simulink model "Control_Block_2021"  (R2022a)
settings: Solver=FixedStepAuto  StartTime=0.0  StopTime=end_time  FixedStep=dt  RelTol=1e-3
values from neighbouring files (symbols this model uses):
  Area = pi() * r0^2    [Main_PD_Control.m]    (also in Test_code.m; main.m = 1.25663706144e-05; main2.m = 1.25663706144e-05)
  Cd = 0.42    [Main_PD_Control.m]    (also in Test_code.m; main.m = 1.05; main2.m = 1.05)
  dl = l / (N - 1)    (= 0.0102040816327)    [load_parameter.m]    (also in main.m; main2.m; testcode_2d.m = 0.0204081632653)
  dt = 0.01    [Main_PD_Control.m]    (also in Test_code.m; load_parameter.m; main.m; main2.m = 0.001)
  EA = E*A    (= 13.8544236023)    [load_parameter.m]    (also in main.m; main2.m; testcode_2d.m = 10555751.3161)
  EI = E*I    (= 1.73180295029e-05)    [load_parameter.m]    (also in main.m; main2.m; testcode_2d.m = 765.291970414)
  K_d = 10    [Main_PD_Control.m]    (also in Test_code.m = 0; main.m; main2.m)
  K_p = 100    [Main_PD_Control.m]    (also in Test_code.m; main.m = 500; main2.m)
  M = zeros(2*N,2*N)    [load_parameter.m]    (also in main.m; main2.m; testcode_2d.m)
  N = length(old_posi)/2    [BoundryJudge.m]    (also in load_parameter.m = 50; main.m = 50; main2.m = 50; testcode_2d.m = 50)
  q0 = zeros(2*N,1)    [load_parameter.m]    (also in main.m; main2.m; testcode_2d.m = q)
  rho_blood = 1025    [main.m]    (also in main2.m)
  tol = EI / l^2 * 1e-3    (= 6.92721180117e-08)    [load_parameter.m]    (also in main.m; main2.m; testcode_2d.m = 0.765291970414)
settings Model: Creator=zhong  LastModifiedBy=zhong
settings DebuggingCC: UnconnectedInputMsg=warning  UnconnectedOutputMsg=warning  UnconnectedLineMsg=warning  UnderSpecifiedDimensionMsg=error
settings RTWCC: DLArmComputeVersion=19.05

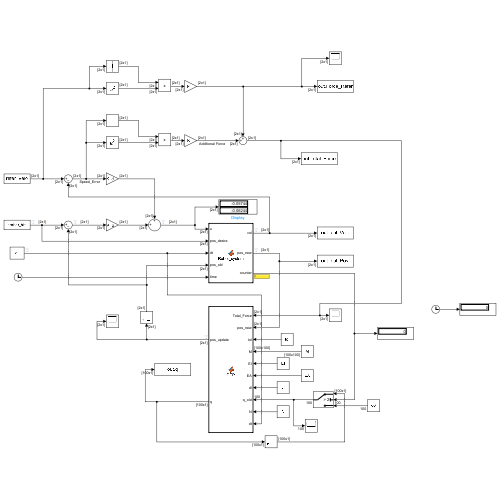
[thumbnail: Simulink's stored preview of the top-level diagram]
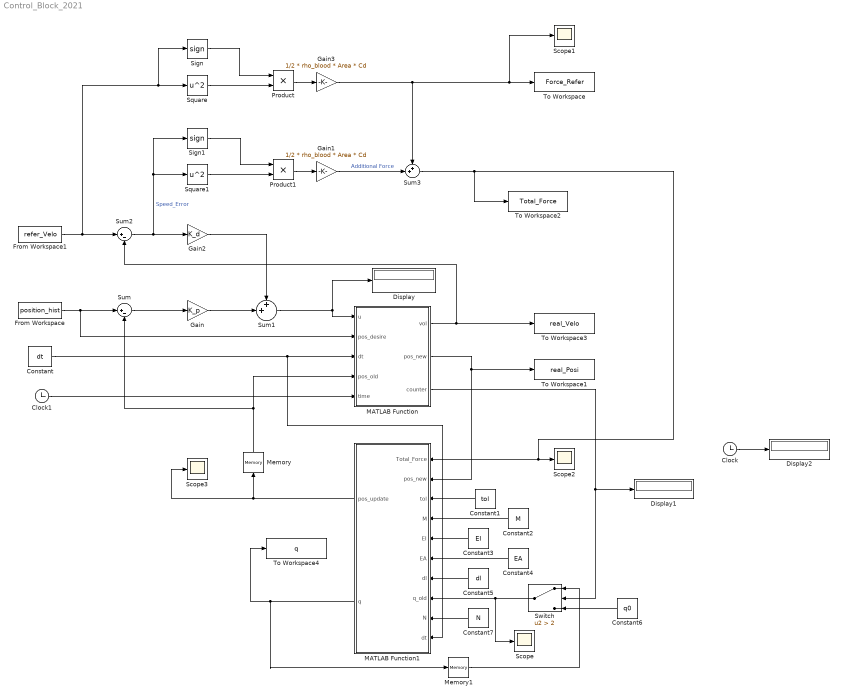
== system Control_Block_2021 ==
  Clock : Clock
  Clock1 : Clock
  Constant : Constant  Value=dt
  Constant1 : Constant  Value=tol
  Constant2 : Constant  Value=M
  Constant3 : Constant  Value=EI
  Constant4 : Constant  Value=EA
  Constant5 : Constant  Value=dl
  Constant6 : Constant  Value=q0
  Constant7 : Constant  Value=N
  Display : Display
  Display1 : Display
  Display2 : Display
  From Workspace : FromWorkspace  VariableName=position_hist
  From Workspace1 : FromWorkspace  VariableName=refer_Velo
  Gain : Gain  Gain=K_p
  Gain1 : Gain  Gain=1/2 * rho_blood * Area * Cd
  Gain2 : Gain  Gain=K_d
  Gain3 : Gain  Gain=1/2 * rho_blood * Area * Cd
  MATLAB Function : MATLAB Function  TreatAsAtomicUnit=on
  MATLAB Function1 : MATLAB Function  TreatAsAtomicUnit=on
  Memory : Memory
  Memory1 : Memory
  Product : Product
  Product1 : Product
  Scope{,1..3} (4 alike) : Scope
  Sign : Signum
  Sign1 : Signum
  Square : Math  Operator=square
  Square1 : Math  Operator=square
  Sum : Sum  Inputs=|+-
  Sum1 : Sum  Inputs=++|
  Sum2 : Sum  Inputs=|+-
  Sum3 : Sum  Inputs=++|
  Switch : Switch  Criteria=u2 > Threshold  Threshold=2  SaturateOnIntegerOverflow=off  InputSameDT=off
  To Workspace : ToWorkspace  VariableName=Force_Refer  SaveFormat=Structure With Time  SampleTime=-1
  To Workspace1 : ToWorkspace  VariableName=real_Posi  SaveFormat=Timeseries  SampleTime=-1
  To Workspace2 : ToWorkspace  VariableName=Total_Force  SaveFormat=Timeseries  SampleTime=-1
  To Workspace3 : ToWorkspace  VariableName=real_Velo  SaveFormat=Timeseries  SampleTime=-1
  To Workspace4 : ToWorkspace  VariableName=q  SaveFormat=Timeseries  SampleTime=-1
  wires:
  From Workspace/1 -> MATLAB Function/2(pos_desire), Sum/1
  Sum/1 -> Gain/1
  Gain/1 -> Sum1/2
  Sum2/1 -> Sign1/1, Square1/1, Gain2/1  "Speed_Error"
  Gain2/1 -> Sum1/1
  Sum1/1 -> Display/1, MATLAB Function/1(u)
  From Workspace1/1 -> Sum2/1, Sign/1, Square/1
  Sum3/1 -> To Workspace2/1, Scope2/1, MATLAB Function1/1(Total_Force)
  Constant/1 -> MATLAB Function1/10(dt), MATLAB Function/3(dt)
  MATLAB Function/2(pos_new) -> MATLAB Function1/2(pos_new), To Workspace1/1
  MATLAB Function/1(vol) -> Sum2/2, To Workspace3/1
  Gain3/1 -> Sum3/1, Scope1/1, To Workspace/1
  Gain1/1 -> Sum3/2  "Additional Force"
  Square/1 -> Product/2
  Sign/1 -> Product/1
  Product/1 -> Gain3/1
  Sign1/1 -> Product1/1
  Square1/1 -> Product1/2
  Product1/1 -> Gain1/1
  MATLAB Function1/1(pos_update) -> Scope3/1, Memory/1
  Constant1/1 -> MATLAB Function1/3(tol)
  Constant2/1 -> MATLAB Function1/4(M)
  Constant3/1 -> MATLAB Function1/5(EI)
  Constant4/1 -> MATLAB Function1/6(EA)
  Constant5/1 -> MATLAB Function1/7(dl)
  Constant7/1 -> MATLAB Function1/9(N)
  Memory/1 -> MATLAB Function/4(pos_old), Sum/2
  MATLAB Function1/2(q) -> Memory1/1, To Workspace4/1
  Switch/1 -> Scope/1, MATLAB Function1/8(q_old)
  Memory1/1 -> Switch/1
  MATLAB Function/3(counter) -> Display1/1, Switch/2
  Clock/1 -> Display2/1
  Clock1/1 -> MATLAB Function/5(time)
  Constant6/1 -> Switch/3

== matlab function Control_Block_2021/MATLAB Function1 ==
  data: Total_Force input; pos_update output; pos_new input; tol input; M input; EI input; EA input; dl input; q_old input; N input; dt input; q output
function [pos_update,q] = DER(Total_Force,pos_new,tol,M,EI,EA,dl,q_old,N,dt)

Ex_force = zeros(2*N,1);

    q = q_old; % Guess
    q(1:2) = pos_new';
    u = (q - q_old) / dt;

    err = 10 * tol;

    % Newton Raphson
    while err > tol

    % Inertia 
    f = M/dt * ((q - q_old) / dt - u);
    J = M/ dt^2;

    % Elastic forces 
    % Linear Spring 
    for k = 1: N-1
        xk = q(2*k-1);
        yk = q(2*k);
        xkp1 = q(2*k+1);
        ykp1 = q(2*k+2); 
        dF = gradEs(xk, yk, xkp1, ykp1, dl, EA);
        dJ = hessEs(xk, yk, xkp1, ykp1, dl, EA);
        f(2*k-1:2*k+2) = f(2*k-1:2*k+2) + dF;
        J(2*k-1:2*k+2, 2*k-1:2*k+2) = ...
        J(2*k-1:2*k+2, 2*k-1:2*k+2) + dJ;
    end

    % Bending spring 
    for k = 2:N-1
        xkm1 = q(2*k-3);
        ykm1 = q(2*k-2);
        xk = q(2*k-1);
        yk = q(2*k);
        xkp1 = q(2*k+1);
        ykp1 = q(2*k+2);
        curvature0 = 0;
        dF = gradEb(xkm1, ykm1, xk, yk, xkp1, ykp1, curvature0, dl, EI);
        dJ = hessEb(xkm1, ykm1, xk, yk, xkp1, ykp1, curvature0, dl, EI);
        f(2*k-3:2*k+2) = f(2*k-3:2*k+2) + dF;
        J(2*k-3:2*k+2, 2*k-3:2*k+2) = ...
            J(2*k-3:2*k+2, 2*k-3:2*k+2) + dJ;
    end
    
    % External force 
    Ex_force(1) = Total_Force(1,:);
    Ex_force(2) = Total_Force(2,:);

    % Weight 
    f = f + Ex_force;

    % Update 
    q(1:(2*N)) = q(1:(2*N)) - J(1:(2*N),1:(2*N)) \ f(1:(2*N));
    err = sum(abs(f(1:(2*N))));
    end

    % Update
%     u = (q - q_old) / dt;
%     q_old = q;

    pos_update = q(1:2,:);
    
%     % plot of sphere position
%     figure(1);
%     plot(result(:,1),result(:,2), 'y');
%     hold on
%     plot(lines(:,1),lines(:,2), 'b');
%     hold on
%     plot(q(1:2:end),q(2:2:end),'ro-');
%     plot(real_Posi(i,1), real_Posi(i,2),'ro');
% %   axis equal
%     axis([-0.5,1.1,-0.1,1.1])
%     hold off
%     drawnow

== matlab function Control_Block_2021/MATLAB Function ==
  data: vol output; u input; pos_desire input; dt input; pos_old input; pos_new output; time input; counter output
function [vol,pos_new,counter] = Robot_system(u,pos_desire,dt,pos_old,time)
pos_new = pos_desire + u;

vol = (pos_new - pos_old)/dt;

counter = time*(1/dt) +1;
% counter = counter + 1;
